simulink model "Simulink_Funktionsblock"  (R2019b)
settings: Solver=VariableStepAuto  StartTime=0.0  StopTime=3000  RelTol=1e-3
values from neighbouring files (symbols this model uses):
  b = double(subs(subs(subs( jacobian(dx_dt,vec_u), vec_x, x_AP), vec_e, e_AP), vec_u, u_AP))    [INIT_Nachbrenner.m]    (also in matlab_workspace.mat = [1 0 0 0 13.4320539233 0 0 0 0.00925048588007 -669669.81608 )
  E = double(subs(subs(subs( jacobian(dx_dt,vec_e), vec_x, x_AP), vec_e, e_AP), vec_u, u_AP))    [INIT_Nachbrenner.m]
  e_AP = [T_bg_in ; T_wt_in ; T_u; ms_bg]    [INIT_Nachbrenner.m]
  g_f = 1    [INIT_Nachbrenner.m]
  k_T = place(lin_A,b,gew_eigenwerte)    [INIT_Nachbrenner.m]
  lin_A = double(subs(subs(subs( jacobian(dx_dt,vec_x), vec_x, x_AP), vec_e, e_AP), vec_u, u_AP))    [INIT_Nachbrenner.m]    (also in matlab_workspace.mat = [-1198.49102382  1040.40539314  157.085630683; 5303.6329886 )
  Par_Ini = [1000;293.15;293.15]    [INIT_Nachbrenner.m]    (also in matlab_workspace.mat = [293.15 293.15 293.15])
  S_v = inv(C_sv*inv(-lin_A+b*k_T)*b)    [INIT_Nachbrenner.m]
  steuerzeit = 500    [INIT_Nachbrenner.m]
  u_AP = [ms_wt_f]    [INIT_Nachbrenner.m]    (also in matlab_workspace.mat = [293.15 293.15 293.15 0.000906192851205 0.000604442426551])
  vec_par = zeros(20,1)    [INIT_Nachbrenner.m]    (also in matlab_workspace.mat = [0.000906192851205 1060.66142274 1060.66142274 0.03280489253)
  x_AP = [double(x_AP_berechnet.x1);double(x_AP_berechnet.x2);double(x_AP_berechnet.x3)]    [INIT_Nachbrenner.m]    (also in matlab_workspace.mat = [900 900 900])
  x_lin_0 = Par_Ini - x_AP    [INIT_Nachbrenner.m]
  y_AP = double(x_AP_berechnet.x2)    [INIT_Nachbrenner.m]
  y_soll = y_AP    [INIT_Nachbrenner.m]
  z = e_AP    [INIT_Nachbrenner.m]
undefined symbols (not defined in the file or in its folder): x_AP_lin
libraries: cstblocks x1
settings Model: Creator=mh981  LastModifiedBy=Vetter
settings DataIOCC: ReturnWorkspaceOutputs=off
settings DebuggingCC: ArithmeticOperatorsInVariantConditions=warning
settings SFSimCC: CustomCodeUndefinedFunction=UseInterfaceOnly

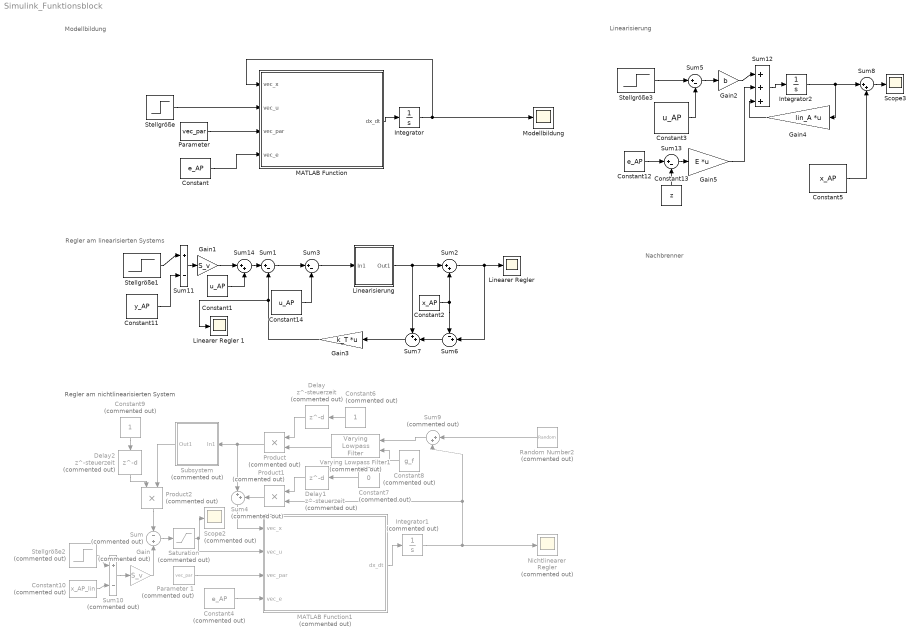
== system Simulink_Funktionsblock ==
  note: Regler am nichtlinearisierten System
  note: Nachbrenner
  note: Regler am linearisierten Systems
  note: Linearisierung
  note: Modellbildung
  Constant : Constant  Value=e_AP
  Constant1 : Constant  Value=u_AP
  Constant10 : Constant  Commented=on  Value=x_AP_lin
  Constant11 : Constant  Value=y_AP
  Constant12 : Constant  Value=e_AP
  Constant13 : Constant  Value=z
  Constant14 : Constant  Value=u_AP
  Constant2 : Constant  Value=x_AP
  Constant3 : Constant  Value=u_AP
  Constant4 : Constant  Commented=on  Value=e_AP
  Constant5 : Constant  Value=x_AP
  Constant6 : Constant  Commented=on
  Constant7 : Constant  Commented=on  Value=0
  Constant8 : Constant  Commented=on  Value=g_f
  Constant9 : Constant  Commented=on
  Delay : Delay  Commented=on  DelayLength=steuerzeit
  Delay1 : Delay  Commented=on  DelayLength=steuerzeit  InitialCondition=1
  Delay2 : Delay  Commented=on  DelayLength=steuerzeit
  Gain : Gain  Commented=on  Gain=S_v
  Gain1 : Gain  Gain=S_v
  Gain2 : Gain  Gain=b
  Gain3 : Gain  Gain=k_T  Multiplication=Matrix(K*u) (u vector)
  Gain4 : Gain  Gain=lin_A  Multiplication=Matrix(K*u) (u vector)
  Gain5 : Gain  Gain=E  Multiplication=Matrix(K*u) (u vector)
  Integrator : Integrator  InitialCondition=Par_Ini
  Integrator1 : Integrator  Commented=on  InitialCondition=Par_Ini
  Integrator2 : Integrator  InitialCondition=x_lin_0
  "Linearer Regler " : Scope
  Linearer Regler 1 : Scope
  "Linearisierung " : Subsystem
  MATLAB Function : MATLAB Function  TreatAsAtomicUnit=on
  MATLAB Function1 : MATLAB Function  Commented=on  TreatAsAtomicUnit=on
  "Modellbildung " : Scope
  Nichtlinearer Regler : Scope  Commented=on
  "Parameter " : Constant  Value=vec_par
  Parameter 1 : Constant  Commented=on  Value=vec_par
  Product : Product  Commented=on
  Product1 : Product  Commented=on
  Product2 : Product  Commented=on
  Random Number2 : RandomNumber  Commented=on  Variance=3  SampleTime=0.1
  Saturation : Saturate  Commented=on  UpperLimit=u_AP*4  LowerLimit=0
  Scope2 : Scope  Commented=on
  Scope3 : Scope
  Stellgröße : Step  Time=2  Before=u_AP  After=u_AP  SampleTime=0
  Stellgröße1 : Step  Time=0  Before=y_soll  After=y_soll  SampleTime=0
  Stellgröße2 : Step  Commented=on  Time=0  Before=u_AP  After=u_AP  SampleTime=0
  Stellgröße3 : Step  Time=0  Before=u_AP  After=u_AP  SampleTime=0
  Subsystem : Subsystem  Commented=on
  Sum : Sum  Commented=on  Inputs=-|+
  Sum{1,3,5,11,13} (5 alike) : Sum  Inputs=|+-
  Sum10 : Sum  Commented=on  Inputs=|+-
  Sum12 : Sum  Inputs=|+++
  Sum14 : Sum  Inputs=|++
  Sum2 : Sum  Inputs=|++
  Sum4 : Sum  Commented=on  Inputs=|++
  Sum6 : Sum  Inputs=-+|
  Sum7 : Sum  Inputs=++|
  Sum8 : Sum  Inputs=|++
  Sum9 : Sum  Commented=on  Inputs=|++
  Varying Lowpass Filter1 : cstblocks/Linear Parameter Varying/Varying Lowpass Filter  Commented=on  N=1
      settings: SourceProductName=Control System Toolbox
  wires:
  MATLAB Function/1(dx_dt) -> Integrator/1
  Stellgröße/1 -> MATLAB Function/2(vec_u)
  "Parameter "/1 -> MATLAB Function/3(vec_par)
  Integrator/1 -> "Modellbildung "/1, MATLAB Function/1(vec_x)
  Constant5/1 -> Sum8/2
  Constant3/1 -> Sum5/2
  Sum8/1 -> Scope3/1
  Stellgröße3/1 -> Sum5/1
  Constant2/1 -> Sum6/1, Sum2/2
  "Linearisierung "/1(Out1) -> Sum7/1, Sum2/1
  Parameter 1/1 -> MATLAB Function1/3(vec_par)
  MATLAB Function1/1(dx_dt) -> Integrator1/1
  Constant/1 -> MATLAB Function/4(vec_e)
  Constant4/1 -> MATLAB Function1/4(vec_e)
  Sum2/1 -> Sum6/2, "Linearer Regler "/1
  Sum6/1 -> Sum7/2
  Sum7/1 -> Gain3/1
  Gain3/1 -> Sum1/2, Linearer Regler 1/1
  Integrator1/1 -> Sum9/2, Product1/2, Nichtlinearer Regler/1
  Random Number2/1 -> Sum9/1
  Sum9/1 -> Varying Lowpass Filter1/1
  Constant8/1 -> Varying Lowpass Filter1/2
  Sum4/1 -> MATLAB Function1/1(vec_x)
  Constant6/1 -> Delay/1
  Product/1 -> Sum4/1, Subsystem/1(In1)
  Delay/1 -> Product/1
  Varying Lowpass Filter1/1 -> Product/2
  Delay1/1 -> Product1/1
  Product1/1 -> Sum4/2
  Constant7/1 -> Delay1/1
  Constant9/1 -> Delay2/1
  Product2/1 -> Sum/1
  Delay2/1 -> Product2/1
  Subsystem/1(Out1) -> Product2/2
  Sum/1 -> Saturation/1
  Saturation/1 -> MATLAB Function1/2(vec_u), Scope2/1
  Stellgröße2/1 -> Sum10/1
  Constant10/1 -> Sum10/2
  Sum10/1 -> Gain/1
  Gain/1 -> Sum/2
  Constant11/1 -> Sum11/2
  Stellgröße1/1 -> Sum11/1
  Sum11/1 -> Gain1/1
  Sum5/1 -> Gain2/1
  Gain2/1 -> Sum12/1
  Gain4/1 -> Sum12/3
  Gain5/1 -> Sum12/2
  Sum12/1 -> Integrator2/1
  Integrator2/1 -> Sum8/1, Gain4/1
  Sum13/1 -> Gain5/1
  Constant12/1 -> Sum13/1
  Constant13/1 -> Sum13/2
  Sum1/1 -> Sum3/1
  Constant14/1 -> Sum3/2
  Sum3/1 -> "Linearisierung "/1(In1)
  Gain1/1 -> Sum14/1
  Sum14/1 -> Sum1/1
  Constant1/1 -> Sum14/2

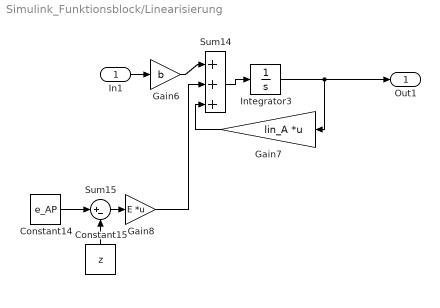
== system Simulink_Funktionsblock/Linearisierung  ==
  In1 : Inport
  Constant14 : Constant  Value=e_AP
  Constant15 : Constant  Value=z
  Gain6 : Gain  Gain=b
  Gain7 : Gain  Gain=lin_A  Multiplication=Matrix(K*u) (u vector)
  Gain8 : Gain  Gain=E  Multiplication=Matrix(K*u) (u vector)
  Integrator3 : Integrator  InitialCondition=x_lin_0
  Sum14 : Sum  Inputs=|+++
  Sum15 : Sum  Inputs=|+-
  Out1 : Outport
  wires:
  Sum14/1 -> Integrator3/1
  Gain7/1 -> Sum14/3
  Gain8/1 -> Sum14/2
  Constant15/1 -> Sum15/2
  Constant14/1 -> Sum15/1
  In1/1 -> Gain6/1
  Sum15/1 -> Gain8/1
  Gain6/1 -> Sum14/1
  Integrator3/1 -> Out1/1, Gain7/1

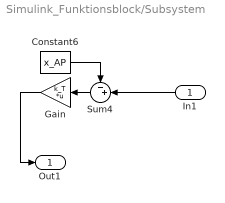
== system Simulink_Funktionsblock/Subsystem ==
  In1 : Inport
  Constant6 : Constant  Value=x_AP
  Gain : Gain  Gain=k_T  Multiplication=Matrix(K*u) (u vector)
  Sum4 : Sum  Inputs=-+|
  Out1 : Outport
  wires:
  Constant6/1 -> Sum4/1
  In1/1 -> Sum4/2
  Sum4/1 -> Gain/1
  Gain/1 -> Out1/1

== matlab function Simulink_Funktionsblock/MATLAB Function1 ==
  data: vec_x input; vec_u input; dx_dt output; vec_par input; vec_e input
%#eml
function dx_dt = Modell_simulink(vec_x ,vec_u , vec_par,vec_e)

dx_dt = Modellgleichung (vec_x ,vec_u , vec_par, vec_e);

== matlab function Simulink_Funktionsblock/MATLAB Function ==
  data: vec_x input; vec_u input; dx_dt output; vec_par input; vec_e input
%#eml
function dx_dt = Modell_simulink(vec_x ,vec_u , vec_par, vec_e)

dx_dt = Modellgleichung (vec_x ,vec_u , vec_par, vec_e);
